simulink model "ETCio100_example"  (Simulink 9.2)
settings: Solver=FixedStepDiscrete  StartTime=0.0  StopTime=inf  FixedStep=1e-3  RelTol=1e-3
undefined symbols (not defined in the file): etcio100_slave
libraries: simulink x1, etherlab_lib x1
settings Model: Creator=juergens  LastModifiedBy=schappler  SimulationMode=external
settings DataIOCC: LimitDataPoints=off  SaveFormat=Dataset  SignalLoggingSaveFormat=Dataset  SaveOutput=off  SignalLogging=off  SaveTime=off
settings OptimizationCC: BlockReduction=off  ConditionallyExecuteInputs=off  OptimizeBlockIOStorage=off  BufferReuse=off  GlobalBufferReuse=off  ExpressionFolding=off  LocalBlockOutputs=off  LifeSpan=auto  OptimizeDataStoreBuffers=off  BusAssignmentInplaceUpdate=off
settings DebuggingCC: UnderspecifiedInitializationDetection=Simplified  MergeDetectMultiDrivingBlocksExec=error  FcnCallInpInsideContextMsg=error  StateNameClashWarn=none  SFUnexpectedBacktrackingDiag=error  SFNoUnconditionalDefaultTransitionDiag=error  SFExecutionAtInitializationDiag=warning
settings HardwareCC: ProdBitPerPointer=64  ProdBitPerSizeT=64  ProdBitPerPtrDiffT=64  ProdLargestAtomicFloat=Float  ProdIntDivRoundTo=Zero  ProdEndianess=LittleEndian  ProdWordSize=64  ProdHWDeviceType=Intel->x86-64 (Windows64)
settings ModelReferenceCC: PropagateSignalLabelsOutOfModel=on
settings RTWCC: SystemTargetFile=etherlab.tlc  TemplateMakefile=etherlab_hrt.tmf  Description=EtherLab PREEMT_RT Real-Time Target
settings STFCustomTargetCC: TargetLangStandard=C99 (ISO)  SystemTargetFile=etherlab.tlc
settings GRTTargetCC: TargetLangStandard=C99 (ISO)  ParMdlRefBuildCompliant=off  CompOptLevelCompliant=off  ConcurrentExecutionCompliant=off  GeneratePreprocessorConditionals=Use local settings  MatFileLogging=off  CPPClassGenCompliant=off  UseToolchainInfoCompliant=off  ExtMode=on  ExtModeStaticAlloc=on  ExtModeStaticAllocSize=10000000  ExtModeMexArgs='10.144.130.83' 0 17725  RTWCAPISignals=on  RTWCAPIParams=on
settings CustomProperty: DataType=int32  Value=2
settings ConfigComp: CovMetricSettings=dwe  CovHtmlReporting=off  CovSaveCumulativeToWorkspaceVar=off  CovSaveSingleToWorkspaceVar=off  CovExternalEMLEnable=on

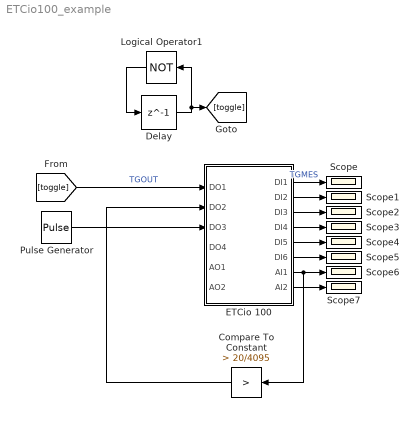
== system ETCio100_example ==
  Compare To Constant : simulink/Logic and Bit Operations/Compare To Constant  relop=>  const=20/4095  OutDataTypeStr=boolean
  Delay : Delay  DelayLength=1
  ETCio 100 : Subsystem
  Logical Operator1 : Logic  Operator=NOT  AllPortsSameDT=off  OutDataTypeStr=boolean
  Pulse Generator : DiscretePulseGenerator  Period=100  SampleTime=-1
  Scope{,1..7} (8 alike) : Scope
  wires:
  ETCio 100/1(DI1) -> Scope/1  "TGMES"
  ETCio 100/2(DI2) -> Scope1/1
  ETCio 100/3(DI3) -> Scope2/1
  ETCio 100/4(DI4) -> Scope3/1
  ETCio 100/5(DI5) -> Scope4/1
  ETCio 100/6(DI6) -> Scope5/1
  ETCio 100/7(AI1) -> Compare To Constant/1, Scope6/1
  ETCio 100/8(AI2) -> Scope7/1
  [toggle] -> ETCio 100/1("DO1  ")  "TGOUT"
  Pulse Generator/1 -> ETCio 100/3("DO3 ")
  Compare To Constant/1 -> ETCio 100/2("DO2 ")
  Delay/1 -> [toggle], Logical Operator1/1
  Logical Operator1/1 -> Delay/1

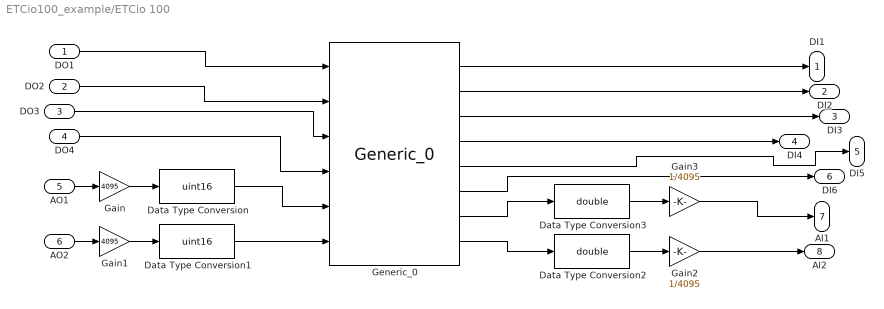
== system ETCio100_example/ETCio 100 ==
  "DO1  " : Inport
  "DO2 " : Inport  Port=2
  "DO3 " : Inport  Port=3
  DO4 : Inport  Port=4
  AO1 : Inport  Port=5
  AO2 : Inport  Port=6
  Data Type Conversion : DataTypeConversion  OutDataTypeStr=uint16
  Data Type Conversion1 : DataTypeConversion  OutDataTypeStr=uint16
  Data Type Conversion2 : DataTypeConversion  OutDataTypeStr=double
  Data Type Conversion3 : DataTypeConversion  OutDataTypeStr=double
  Gain : Gain  Gain=4095
  Gain1 : Gain  Gain=4095
  Gain2 : Gain  Gain=1/4095
  Gain3 : Gain  Gain=1/4095
  Generic_0 : etherlab_lib/EtherCAT/Generic_0  master=0  index=0  rv=etcio100_slave()  param=[]  tsample=-1  debug=0
  DI1 : Outport
  DI2 : Outport  Port=2
  DI3 : Outport  Port=3
  DI4 : Outport  Port=4
  DI5 : Outport  Port=5
  DI6 : Outport  Port=6
  AI1 : Outport  Port=7
  AI2 : Outport  Port=8
  wires:
  "DO1  "/1 -> Generic_0/1
  Generic_0/1 -> DI1/1
  Generic_0/3 -> DI3/1
  "DO3 "/1 -> Generic_0/3
  Generic_0/5 -> DI5/1
  DO4/1 -> Generic_0/4
  "DO2 "/1 -> Generic_0/2
  Generic_0/2 -> DI2/1
  Data Type Conversion/1 -> Generic_0/5
  Generic_0/6 -> DI6/1
  Data Type Conversion1/1 -> Generic_0/6
  Generic_0/7 -> Data Type Conversion3/1
  Gain2/1 -> AI2/1
  Generic_0/8 -> Data Type Conversion2/1
  Gain3/1 -> AI1/1
  Generic_0/4 -> DI4/1
  AO1/1 -> Gain/1
  AO2/1 -> Gain1/1
  Data Type Conversion2/1 -> Gain2/1
  Data Type Conversion3/1 -> Gain3/1
  Gain/1 -> Data Type Conversion/1
  Gain1/1 -> Data Type Conversion1/1
